simulink subsystem "BAM_Controller"  (R2026a)
settings: Solver=VariableStepAuto
undefined symbols (not defined in the file): DiscIntNeverNeededParam, SimIn, SimPar
libraries: simulink x11, starslibMathOperations x2, sharedTrackingLibrary x1, simulink_extras x1, starslibAxisTransformations x1
(part 2 of 3)

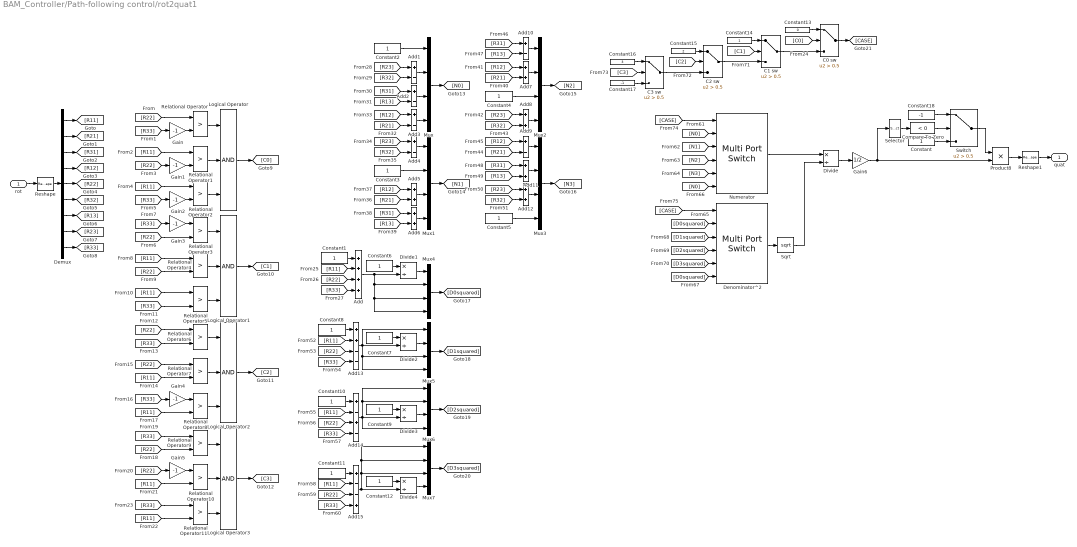
== system BAM_Controller/Path-following control/rot2quat1 ==
  rot : Inport
  Add : Sum  Inputs=++++
  Add{1..4,9..10} (6 alike) : Sum  Inputs=+-
  Add{5..8,11..12} (6 alike) : Sum
  Add13 : Sum  Inputs=++--
  Add14 : Sum  Inputs=+-+-
  Add15 : Sum  Inputs=+--+
  C0 sw : Switch  Criteria=u2 > Threshold  Threshold=0.5  SaturateOnIntegerOverflow=off  InputSameDT=off
  C1 sw : Switch  Criteria=u2 > Threshold  Threshold=0.5  SaturateOnIntegerOverflow=off  InputSameDT=off
  C2 sw : Switch  Criteria=u2 > Threshold  Threshold=0.5  SaturateOnIntegerOverflow=off  InputSameDT=off
  C3 sw : Switch  Criteria=u2 > Threshold  Threshold=0.5  SaturateOnIntegerOverflow=off  InputSameDT=off
  Compare To Zero : simulink/Logic and Bit Operations/Compare To Zero  relop=<  OutDataTypeStr=boolean
  Constant{,1..12,14} (14 alike) : Constant
  Constant13 : Constant  Value=0
  Constant15 : Constant  Value=2
  Constant16 : Constant  Value=3
  Constant17 : Constant  Value=-1
  Constant18 : Constant  Value=-1
  Demux : Demux  Outputs=9
  Denominator^2 : MultiPortSwitch  DataPortOrder=Zero-based contiguous  Inputs=4  DataPortForDefault=Additional data port  zeroidx=on  SaturateOnIntegerOverflow=off  InputSameDT=off
  Divide{,1..4} (5 alike) : Product  Inputs=*/
  Gain{,1..5} (6 alike) : Gain  Gain=-1
  Gain6 : Gain  Gain=1/2
  Logical Operator{,1..3} (4 alike) : Logic  Inputs=3  AllPortsSameDT=off  OutDataTypeStr=boolean
  Mux{,1..7} (8 alike) : Mux
  Numerator : MultiPortSwitch  DataPortOrder=Zero-based contiguous  Inputs=4  DataPortForDefault=Additional data port  zeroidx=on  SaturateOnIntegerOverflow=off  InputSameDT=off
  Product8 : Product
  Relational Operator{,1..11} (12 alike) : RelationalOperator  Operator=>  OutDataTypeStr=boolean  RndMeth=Simplest  InputSameDT=off
  Reshape : Reshape  OutputDimensionality=Column vector (2-D)
  Reshape1 : Reshape  OutputDimensionality=Column vector (2-D)
  Selector : Selector  InputPortWidth=4  IndexOptions=Index vector (dialog)  Indices=1  OutputSizes=1
  Sqrt : Sqrt
  Switch : Switch  Criteria=u2 > Threshold  Threshold=0.5  SaturateOnIntegerOverflow=off  InputSameDT=off
  quat : Outport  VectorParamsAs1DForOutWhenUnconnected=off
  wires:
  Product8/1 -> Reshape1/1
  Reshape1/1 -> quat/1
  Selector/1 -> Compare To Zero/1
  Compare To Zero/1 -> Switch/2
  Constant18/1 -> Switch/1
  Constant/1 -> Switch/3
  Switch/1 -> Product8/1
  [R23] -> Add1/1
  Add/1 -> Divide1/2, Mux4/2, Mux4/3, Mux4/4
  Divide1/1 -> Mux4/1
  Divide2/1 -> Mux5/2
  [N0] -> Numerator/6
  C2 sw/1 -> C1 sw/3
  Constant6/1 -> Divide1/1
  [R12] -> Add7/1
  Constant17/1 -> C3 sw/3
  [N3] -> Numerator/5
  Mux1/1 -> [N1]
  Add7/1 -> Mux2/2
  [N0] -> Numerator/2
  Constant14/1 -> C1 sw/1
  [R21] -> Add3/2
  [R21] -> Add7/2
  [R12] -> Add5/1
  Gain3/1 -> Relational Operator3/1
  Gain5/1 -> Relational Operator10/1
  [R33] -> Relational Operator9/1
  Relational Operator10/1 -> Logical Operator3/2
  Denominator^2/1 -> Sqrt/1
  [R33] -> Gain/1
  Logical Operator/1 -> [C0]
  [R11] -> Relational Operator5/1
  [R11] -> Relational Operator4/1
  [R22] -> Relational Operator/1
  Demux/6 -> [R32]
  Relational Operator4/1 -> Logical Operator1/2
  Relational Operator2/1 -> Logical Operator/3
  [R33] -> Relational Operator5/2
  [R22] -> Relational Operator9/2
  [R22] -> Relational Operator4/2
  Relational Operator9/1 -> Logical Operator3/1
  Demux/4 -> [R12]
  Demux/3 -> [R31]
  Relational Operator5/1 -> Logical Operator1/3
  Numerator/1 -> Divide/1
  Gain4/1 -> Relational Operator8/1
  Divide/1 -> Gain6/1
  Relational Operator8/1 -> Logical Operator2/3
  [R11] -> Relational Operator2/1
  Relational Operator/1 -> Logical Operator/1
  [R33] -> Gain4/1
  [R22] -> Relational Operator3/2
  Gain1/1 -> Relational Operator1/2
  Relational Operator1/1 -> Logical Operator/2
  Reshape/1 -> Demux/1
  [R33] -> Gain3/1
  Demux/5 -> [R22]
  Demux/8 -> [R23]
  C1 sw/1 -> C0 sw/3
  Constant13/1 -> C0 sw/1
  Divide4/1 -> Mux7/4
  Constant4/1 -> Mux2/3
  [D2squared] -> Denominator^2/4
  [R32] -> Add12/2
  [R23] -> Add12/1
  Sqrt/1 -> Divide/2
  [R13] -> Add2/2
  Demux/1 -> [R11]
  Relational Operator3/1 -> Logical Operator1/1
  Demux/2 -> [R21]
  Add12/1 -> Mux3/3
  [R11] -> Relational Operator11/2
  Relational Operator11/1 -> Logical Operator3/3
  [R22] -> Gain5/1
  [R33] -> Gain2/1
  [R11] -> Relational Operator10/2
  Logical Operator1/1 -> [C1]
  Logical Operator2/1 -> [C2]
  [R33] -> Relational Operator6/2
  [R33] -> Relational Operator11/1
  [R22] -> Relational Operator6/1
  [R32] -> Add4/2
  [R22] -> Gain1/1
  [R23] -> Add4/1
  [CASE] -> Denominator^2/1
  Add4/1 -> Mux1/1
  Relational Operator6/1 -> Logical Operator2/1
  [D0squared] -> Denominator^2/2
  Demux/9 -> [R33]
  [D1squared] -> Denominator^2/3
  [R11] -> Add15/2
  Mux2/1 -> [N2]
  Demux/7 -> [R13]
  Constant11/1 -> Add15/1
  [R11] -> Relational Operator7/2
  Logical Operator3/1 -> [C3]
  Mux7/1 -> [D3squared]
  [D3squared] -> Denominator^2/5
  [R11] -> Relational Operator8/2
  [R22] -> Relational Operator7/1
  Gain/1 -> Relational Operator/2
  [R33] -> Add15/4
  [R22] -> Add15/3
  Constant12/1 -> Divide4/1
  [R22] -> Add/3
  Constant3/1 -> Mux1/2
  [R11] -> Relational Operator1/1
  Relational Operator7/1 -> Logical Operator2/2
  [R12] -> Add3/1
  Add6/1 -> Mux1/4
  Add3/1 -> Mux/4
  [R13] -> Add6/2
  [R31] -> Add6/1
  [N1] -> Numerator/3
  rot/1 -> Reshape/1
  Mux4/1 -> [D0squared]
  Gain2/1 -> Relational Operator2/2
  [C0] -> C0 sw/2
  [C2] -> C2 sw/2
  C3 sw/1 -> C2 sw/3
  Constant16/1 -> C3 sw/1
  Constant15/1 -> C2 sw/1
  Divide3/1 -> Mux6/3
  Add15/1 -> Divide4/2, Mux7/3, Mux7/2, Mux7/1
  [CASE] -> Numerator/1
  Constant9/1 -> Divide3/1
  [R11] -> Add13/2
  [R11] -> Add14/2
  Add1/1 -> Mux/2
  Add14/1 -> Divide3/2, Mux6/4, Mux6/2, Mux6/1
  Mux6/1 -> [D2squared]
  [R22] -> Add14/3
  [R22] -> Add13/3
  [R33] -> Add14/4
  [R33] -> Add/4
  Constant10/1 -> Add14/1
  [R32] -> Add1/2
  Mux/1 -> [N0]
  Constant8/1 -> Add13/1
  [R33] -> Add13/4
  [R11] -> Add/2
  C0 sw/1 -> [CASE]
  Add10/1 -> Mux2/1
  [R13] -> Add10/2
  [R21] -> Add5/2
  [C3] -> C3 sw/2
  Add5/1 -> Mux1/3
  [R31] -> Add2/1
  [R31] -> Add10/1
  [N2] -> Numerator/4
  Constant7/1 -> Divide2/1
  Mux5/1 -> [D1squared]
  [D0squared] -> Denominator^2/6
  Add13/1 -> Divide2/2, Mux5/1, Mux5/3, Mux5/4
  [R21] -> Add9/2
  [C1] -> C1 sw/2
  Gain6/1 -> Selector/1, Product8/2
  Constant2/1 -> Mux/1
  Add9/1 -> Mux3/1
  [R12] -> Add9/1
  [R32] -> Add8/2
  Add8/1 -> Mux2/4
  Add11/1 -> Mux3/2
  [R13] -> Add11/2
  Mux3/1 -> [N3]
  Add2/1 -> Mux/3
  [R23] -> Add8/1
  Constant1/1 -> Add/1
  Constant5/1 -> Mux3/4
  [R31] -> Add11/1

== system BAM_Controller/PI&FF Rate Controller/Gain Kff/Diagonalize Vector ==
  Vector : Inport
  Constant2 : Constant  Value=0
  Demux : Demux  Outputs=3
  Reshape (9) to [3x3] column-major : Reshape  OutputDimensionality=Customize  OutputDimensions=[3,3]
  Vector Concatenate : Concatenate  NumInputs=9
  Matrix : Outport  VectorParamsAs1DForOutWhenUnconnected=off
  wires:
  Demux/3 -> Vector Concatenate/9
  Demux/2 -> Vector Concatenate/5
  Vector Concatenate/1 -> Reshape (9) to [3x3] column-major/1
  Reshape (9) to [3x3] column-major/1 -> Matrix/1
  Demux/1 -> Vector Concatenate/1
  Constant2/1 -> Vector Concatenate/3, Vector Concatenate/4, Vector Concatenate/6, Vector Concatenate/7, Vector Concatenate/8, Vector Concatenate/2
  Vector/1 -> Demux/1

== system BAM_Controller/PI&FF Rate Controller/Gain Ki/Diagonalize Vector ==
  Vector : Inport
  Constant2 : Constant  Value=0
  Demux : Demux  Outputs=3
  Reshape (9) to [3x3] column-major : Reshape  OutputDimensionality=Customize  OutputDimensions=[3,3]
  Vector Concatenate : Concatenate  NumInputs=9
  Matrix : Outport  VectorParamsAs1DForOutWhenUnconnected=off
  wires:
  Demux/3 -> Vector Concatenate/9
  Demux/2 -> Vector Concatenate/5
  Vector Concatenate/1 -> Reshape (9) to [3x3] column-major/1
  Reshape (9) to [3x3] column-major/1 -> Matrix/1
  Demux/1 -> Vector Concatenate/1
  Constant2/1 -> Vector Concatenate/3, Vector Concatenate/4, Vector Concatenate/6, Vector Concatenate/7, Vector Concatenate/8, Vector Concatenate/2
  Vector/1 -> Demux/1

== system BAM_Controller/PI&FF Rate Controller/Gain Kp/Diagonalize Vector ==
  Vector : Inport
  Constant2 : Constant  Value=0
  Demux : Demux  Outputs=3
  Reshape (9) to [3x3] column-major : Reshape  OutputDimensionality=Customize  OutputDimensions=[3,3]
  Vector Concatenate : Concatenate  NumInputs=9
  Matrix : Outport  VectorParamsAs1DForOutWhenUnconnected=off
  wires:
  Demux/3 -> Vector Concatenate/9
  Demux/2 -> Vector Concatenate/5
  Vector Concatenate/1 -> Reshape (9) to [3x3] column-major/1
  Reshape (9) to [3x3] column-major/1 -> Matrix/1
  Demux/1 -> Vector Concatenate/1
  Constant2/1 -> Vector Concatenate/3, Vector Concatenate/4, Vector Concatenate/6, Vector Concatenate/7, Vector Concatenate/8, Vector Concatenate/2
  Vector/1 -> Demux/1

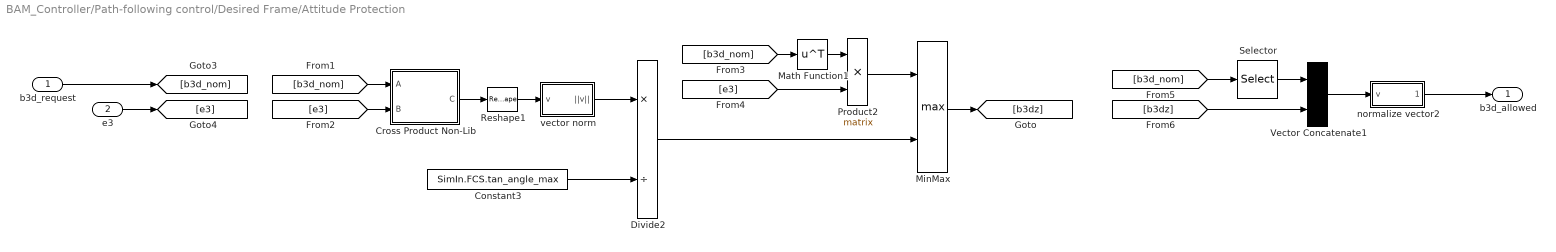
== system BAM_Controller/Path-following control/Desired Frame/Attitude Protection ==
  b3d_request : Inport
  e3 : Inport  Port=2
  Constant3 : Constant  Value=SimIn.FCS.tan_angle_max
  Cross Product Non-Lib : Subsystem
  Divide2 : Product  Inputs=*/
  Math Function1 : Math  Operator=transpose  SignedPower=on
  MinMax : MinMax  Function=max  Inputs=2
  Product2 : Product  Multiplication=Matrix(*)
  Reshape1 : Reshape  OutputDimensionality=Column vector (2-D)
  Selector : Selector  InputPortWidth=3  IndexOptions=Index vector (dialog)  Indices=[1 2]  OutputSizes=1
  Vector Concatenate1 : Concatenate  Mode=Multidimensional array
  normalize vector2 : Subsystem
  vector norm : Subsystem
  b3d_allowed : Outport  VectorParamsAs1DForOutWhenUnconnected=off
  wires:
  MinMax/1 -> [b3dz]
  [e3] -> Product2/2
  Divide2/1 -> MinMax/2
  Product2/1 -> MinMax/1
  Constant3/1 -> Divide2/2
  [e3] -> Cross Product Non-Lib/2(B)
  [b3d_nom] -> Cross Product Non-Lib/1(A)
  Reshape1/1 -> vector norm/1(v)
  vector norm/1(||v||) -> Divide2/1
  normalize vector2/1(v / ||v||) -> b3d_allowed/1
  Cross Product Non-Lib/1(C) -> Reshape1/1
  [b3d_nom] -> Selector/1
  Selector/1 -> Vector Concatenate1/1
  Vector Concatenate1/1 -> normalize vector2/1(v)
  [b3dz] -> Vector Concatenate1/2
  b3d_request/1 -> [b3d_nom]
  e3/1 -> [e3]
  Math Function1/1 -> Product2/1
  [b3d_nom] -> Math Function1/1

== system BAM_Controller/Path-following control/Desired Frame/Cross Product Non-Lib ==
  A : Inport
  B : Inport  Port=2
  Subsystem : Subsystem
  Subsystem1 : Subsystem
  Sum : Sum  Inputs=+|-  InputSameDT=on  SaturateOnIntegerOverflow=on  OutDataTypeStr=Inherit: Same as first input
  C : Outport  VectorParamsAs1DForOutWhenUnconnected=off
  wires:
  Subsystem/1(Out1) -> Sum/1
  B/1 -> Subsystem/2(B), Subsystem1/2(B)
  Subsystem1/1(Out1) -> Sum/2
  A/1 -> Subsystem/1(A), Subsystem1/1(A)
  Sum/1 -> C/1

== system BAM_Controller/Path-following control/Desired Frame/DLPF ==
  In1 : Inport
  Constant1 : Constant  Value=0
  Discrete-Time Integrator1 : DiscreteIntegrator  gainval=1  ExternalReset=either  InitialConditionSource=external  SampleTime=SimIn.FCS.t_control  UpperSaturationLimit=1  LowerSaturationLimit=0  ICPrevOutput=DiscIntNeverNeededParam  ICPrevScaledInput=DiscIntNeverNeededParam
  Gain : Gain  Gain=w
  Sum : Sum  Inputs=|+-
  Out1 : Outport  VectorParamsAs1DForOutWhenUnconnected=off
  wires:
  In1/1 -> Discrete-Time Integrator1/3, Sum/1
  Sum/1 -> Gain/1
  Discrete-Time Integrator1/1 -> Out1/1, Sum/2
  Constant1/1 -> Discrete-Time Integrator1/2
  Gain/1 -> Discrete-Time Integrator1/1

== system BAM_Controller/Path-following control/Desired Frame/DLPF1 ==
  In1 : Inport
  Constant1 : Constant  Value=0
  Discrete-Time Integrator1 : DiscreteIntegrator  gainval=1  ExternalReset=either  InitialConditionSource=external  SampleTime=SimIn.FCS.t_control  UpperSaturationLimit=1  LowerSaturationLimit=0  ICPrevOutput=DiscIntNeverNeededParam  ICPrevScaledInput=DiscIntNeverNeededParam
  Gain : Gain  Gain=w
  Sum : Sum  Inputs=|+-
  Out1 : Outport  VectorParamsAs1DForOutWhenUnconnected=off
  wires:
  Gain/1 -> Discrete-Time Integrator1/1
  Constant1/1 -> Discrete-Time Integrator1/2
  Discrete-Time Integrator1/1 -> Sum/2, Out1/1
  Sum/1 -> Gain/1
  In1/1 -> Sum/1, Discrete-Time Integrator1/3

== system BAM_Controller/Path-following control/Desired Frame/normalize vector1 ==
  v : Inport
  Add : Sum
  Compare To Constant : simulink/Logic and Bit Operations/Compare To Constant  relop===  const=0  OutDataTypeStr=boolean
  Constant : Constant
  Constant1 : Constant  Value=0
  Divide3 : Product  Inputs=*/
  Switch : Switch  Criteria=u2 > Threshold  Threshold=0.5  SaturateOnIntegerOverflow=off  InputSameDT=off
  vector norm : Subsystem
  v / ||v|| : Outport  VectorParamsAs1DForOutWhenUnconnected=off
  wires:
  Divide3/1 -> v / ||v||/1
  vector norm/1(||v||) -> Compare To Constant/1, Add/1
  v/1 -> vector norm/1(v), Divide3/1
  Add/1 -> Divide3/2
  Switch/1 -> Add/2
  Compare To Constant/1 -> Switch/2
  Constant/1 -> Switch/1
  Constant1/1 -> Switch/3

== system BAM_Controller/Path-following control/Desired Frame/normalize vector2 ==
  v : Inport
  Add : Sum
  Compare To Constant : simulink/Logic and Bit Operations/Compare To Constant  relop===  const=0  OutDataTypeStr=boolean
  Constant : Constant
  Constant1 : Constant  Value=0
  Divide3 : Product  Inputs=*/
  Switch : Switch  Criteria=u2 > Threshold  Threshold=0.5  SaturateOnIntegerOverflow=off  InputSameDT=off
  vector norm : Subsystem
  v / ||v|| : Outport  VectorParamsAs1DForOutWhenUnconnected=off
  wires:
  Constant1/1 -> Switch/3
  Constant/1 -> Switch/1
  Compare To Constant/1 -> Switch/2
  Switch/1 -> Add/2
  Add/1 -> Divide3/2
  v/1 -> Divide3/1, vector norm/1(v)
  vector norm/1(||v||) -> Add/1, Compare To Constant/1
  Divide3/1 -> v / ||v||/1

== system BAM_Controller/Path-following control/Path/DLPF7 ==
  x : Inport
  Discrete-Time Integrator : DiscreteIntegrator  InitialConditionSource=external  SampleTime=-1  ICPrevOutput=DiscIntNeverNeededParam  ICPrevScaledInput=DiscIntNeverNeededParam
  Gain : Gain  Gain=bw
  Sum : Sum  Inputs=-+|
  xf : Outport  VectorParamsAs1DForOutWhenUnconnected=off
  wires:
  x/1 -> Discrete-Time Integrator/2, Sum/2
  Sum/1 -> Gain/1
  Gain/1 -> Discrete-Time Integrator/1
  Discrete-Time Integrator/1 -> Sum/1, xf/1

== system BAM_Controller/Path-following control/Path/DLPF8 ==
  x : Inport
  Discrete-Time Integrator : DiscreteIntegrator  InitialConditionSource=external  SampleTime=-1  ICPrevOutput=DiscIntNeverNeededParam  ICPrevScaledInput=DiscIntNeverNeededParam
  Gain : Gain  Gain=bw
  Sum : Sum  Inputs=-+|
  xf : Outport  VectorParamsAs1DForOutWhenUnconnected=off
  wires:
  Discrete-Time Integrator/1 -> xf/1, Sum/1
  Gain/1 -> Discrete-Time Integrator/1
  Sum/1 -> Gain/1
  x/1 -> Sum/2, Discrete-Time Integrator/2

== system BAM_Controller/Path-following control/Path/Heading Hold Logic prevents badness when trajectory is vertical ==
  quat : Inport
  tangent : Inport  Port=2
  Constant1 : Constant  Value=SimIn.FCS.e3
  Constant3 : Constant  Value=0.05
  Cross Product1 : starslibMathOperations/Cross Product
  Heading Vector in Horz Plane : Subsystem
  Relational Operator : RelationalOperator  Operator=>  OutDataTypeStr=boolean  RndMeth=Simplest  InputSameDT=off
  Vector Norm : Subsystem  mask(Vector Norm){}
      mask help: Calculates the 2-norm of the input vector.
      settings: CopyFcn=set_param(gcb,'LinkStatus','none')
  tangentDes3 : Switch  Criteria=u2 > Threshold  Threshold=0.5  SaturateOnIntegerOverflow=off  InputSameDT=off
  t_F : Outport  VectorParamsAs1DForOutWhenUnconnected=off
  wires:
  Relational Operator/1 -> tangentDes3/2
  [headingVector] -> tangentDes3/3
  Constant3/1 -> Relational Operator/2
  Vector Norm/1(||v||) -> Relational Operator/1
  Constant1/1 -> Cross Product1/2
  Cross Product1/1 -> Vector Norm/1(v)
  tangent/1 -> tangentDes3/1, Cross Product1/1
  tangentDes3/1 -> t_F/1
  Heading Vector in Horz Plane/1(headVec) -> [headingVector]
  quat/1 -> Heading Vector in Horz Plane/1(quat)

== system BAM_Controller/Path-following control/Path/normalize vector2 ==
  v : Inport
  Add : Sum
  Compare To Constant : simulink/Logic and Bit Operations/Compare To Constant  relop===  const=0  OutDataTypeStr=boolean
  Constant : Constant
  Constant1 : Constant  Value=0
  Divide3 : Product  Inputs=*/
  Switch : Switch  Criteria=u2 > Threshold  Threshold=0.5  SaturateOnIntegerOverflow=off  InputSameDT=off
  vector norm : Subsystem
  v / ||v|| : Outport  VectorParamsAs1DForOutWhenUnconnected=off
  wires:
  Divide3/1 -> v / ||v||/1
  vector norm/1(||v||) -> Compare To Constant/1, Add/1
  v/1 -> vector norm/1(v), Divide3/1
  Add/1 -> Divide3/2
  Switch/1 -> Add/2
  Compare To Constant/1 -> Switch/2
  Constant/1 -> Switch/1
  Constant1/1 -> Switch/3

== system BAM_Controller/Path-following control/f_c/prevent div by 0 ==
  In1 : Inport
  Compare To Zero : simulink/Logic and Bit Operations/Compare To Zero  relop=~=  OutDataTypeStr=boolean
  Constant : Constant
  Switch : Switch  Criteria=u2 > Threshold  SaturateOnIntegerOverflow=off  InputSameDT=off
  Out1 : Outport  VectorParamsAs1DForOutWhenUnconnected=off
  wires:
  Switch/1 -> Out1/1
  Constant/1 -> Switch/3
  Compare To Zero/1 -> Switch/2
  In1/1 -> Switch/1, Compare To Zero/1

== system BAM_Controller/Path-following control/omega_c/Subsystem ==
  function : TriggerPort  TriggerType=function-call  VariantControl=(inherit)
  From : From  Commented=on  GotoTag=Rtilde
  Gain2 : Gain  Commented=on  Gain=SimIn.FCS.r2d
  MATLAB Function : MATLAB Function  Commented=on  TreatAsAtomicUnit=on
  desired frame error : Scope  Commented=on
      settings: SampleTime=FCS.t_control  ActiveDisplayYMinimum=-0.00376  ActiveDisplayYMaximum=0.00938  DataLoggingVariableName=ScopeData2
  wires:
  Gain2/1 -> desired frame error/1
  From/1 -> MATLAB Function/1(R)
  MATLAB Function/1(rpy) -> Gain2/1

== system BAM_Controller/Path-following control/Desired Frame/Attitude Protection/Cross Product Non-Lib ==
  A : Inport
  B : Inport  Port=2
  Subsystem : Subsystem
  Subsystem1 : Subsystem
  Sum : Sum  Inputs=+|-  InputSameDT=on  SaturateOnIntegerOverflow=on  OutDataTypeStr=Inherit: Same as first input
  C : Outport  VectorParamsAs1DForOutWhenUnconnected=off
  wires:
  Subsystem/1(Out1) -> Sum/1
  B/1 -> Subsystem/2(B), Subsystem1/2(B)
  Subsystem1/1(Out1) -> Sum/2
  A/1 -> Subsystem/1(A), Subsystem1/1(A)
  Sum/1 -> C/1

== system BAM_Controller/Path-following control/Desired Frame/Attitude Protection/normalize vector2 ==
  v : Inport
  Add : Sum
  Compare To Constant : simulink/Logic and Bit Operations/Compare To Constant  relop===  const=0  OutDataTypeStr=boolean
  Constant : Constant
  Constant1 : Constant  Value=0
  Divide3 : Product  Inputs=*/
  Switch : Switch  Criteria=u2 > Threshold  Threshold=0.5  SaturateOnIntegerOverflow=off  InputSameDT=off
  vector norm : Subsystem
  v / ||v|| : Outport  VectorParamsAs1DForOutWhenUnconnected=off
  wires:
  Constant1/1 -> Switch/3
  Constant/1 -> Switch/1
  Compare To Constant/1 -> Switch/2
  Switch/1 -> Add/2
  Add/1 -> Divide3/2
  v/1 -> Divide3/1, vector norm/1(v)
  vector norm/1(||v||) -> Add/1, Compare To Constant/1
  Divide3/1 -> v / ||v||/1

== system BAM_Controller/Path-following control/Desired Frame/Attitude Protection/vector norm ==
  v : Inport
  Abs3 : Abs  SaturateOnIntegerOverflow=off
  Math Function1 : Math  Operator=transpose  SignedPower=on
  Matrix Multiply1 : Product  Multiplication=Matrix(*)
  Reshape7 : Reshape  OutputDimensionality=Column vector (2-D)
  Sqrt3 : Sqrt
  ||v|| : Outport  VectorParamsAs1DForOutWhenUnconnected=off
  wires:
  Sqrt3/1 -> ||v||/1
  Abs3/1 -> Sqrt3/1
  v/1 -> Reshape7/1
  Matrix Multiply1/1 -> Abs3/1
  Math Function1/1 -> Matrix Multiply1/1
  Reshape7/1 -> Matrix Multiply1/2, Math Function1/1

== system BAM_Controller/Path-following control/Desired Frame/Cross Product Non-Lib/Subsystem ==
  A : Inport
  B : Inport  Port=2
  Demux : Demux  Outputs=3
  Demux1 : Demux  Outputs=3
  Mux : Mux  Inputs=3
  i x j : Product  InputSameDT=on  SaturateOnIntegerOverflow=on  OutDataTypeStr=Inherit: Same as first input
  j x k : Product  InputSameDT=on  SaturateOnIntegerOverflow=on  OutDataTypeStr=Inherit: Same as first input
  k x i : Product  InputSameDT=on  SaturateOnIntegerOverflow=on  OutDataTypeStr=Inherit: Same as first input
  Out1 : Outport  VectorParamsAs1DForOutWhenUnconnected=off
  wires:
  Demux1/3 -> j x k/2
  i x j/1 -> Mux/3
  Demux/3 -> k x i/1
  Mux/1 -> Out1/1
  Demux/1 -> i x j/1
  A/1 -> Demux/1
  j x k/1 -> Mux/1
  Demux1/1 -> k x i/2
  B/1 -> Demux1/1
  k x i/1 -> Mux/2
  Demux1/2 -> i x j/2
  Demux/2 -> j x k/1

== system BAM_Controller/Path-following control/Desired Frame/Cross Product Non-Lib/Subsystem1 ==
  A : Inport
  B : Inport  Port=2
  Demux : Demux  Outputs=3
  Demux1 : Demux  Outputs=3
  Mux : Mux  Inputs=3
  i x k : Product  InputSameDT=on  SaturateOnIntegerOverflow=on  OutDataTypeStr=Inherit: Same as first input
  j x i : Product  InputSameDT=on  SaturateOnIntegerOverflow=on  OutDataTypeStr=Inherit: Same as first input
  k x j : Product  InputSameDT=on  SaturateOnIntegerOverflow=on  OutDataTypeStr=Inherit: Same as first input
  Out1 : Outport  VectorParamsAs1DForOutWhenUnconnected=off
  wires:
  Demux/1 -> i x k/1
  A/1 -> Demux/1
  j x i/1 -> Mux/3
  Demux1/3 -> i x k/2
  k x j/1 -> Mux/1
  Demux1/1 -> j x i/2
  B/1 -> Demux1/1
  Demux/3 -> k x j/1
  Demux/2 -> j x i/1
  Mux/1 -> Out1/1
  i x k/1 -> Mux/2
  Demux1/2 -> k x j/2

== system BAM_Controller/Path-following control/Desired Frame/normalize vector1/vector norm ==
  v : Inport
  Abs3 : Abs  SaturateOnIntegerOverflow=off
  Math Function1 : Math  Operator=transpose  SignedPower=on
  Matrix Multiply1 : Product  Multiplication=Matrix(*)
  Reshape7 : Reshape  OutputDimensionality=Column vector (2-D)
  Sqrt3 : Sqrt
  ||v|| : Outport  VectorParamsAs1DForOutWhenUnconnected=off
  wires:
  Sqrt3/1 -> ||v||/1
  v/1 -> Reshape7/1
  Matrix Multiply1/1 -> Abs3/1
  Math Function1/1 -> Matrix Multiply1/1
  Abs3/1 -> Sqrt3/1
  Reshape7/1 -> Matrix Multiply1/2, Math Function1/1

== system BAM_Controller/Path-following control/Desired Frame/normalize vector2/vector norm ==
  v : Inport
  Abs3 : Abs  SaturateOnIntegerOverflow=off
  Math Function1 : Math  Operator=transpose  SignedPower=on
  Matrix Multiply1 : Product  Multiplication=Matrix(*)
  Reshape7 : Reshape  OutputDimensionality=Column vector (2-D)
  Sqrt3 : Sqrt
  ||v|| : Outport  VectorParamsAs1DForOutWhenUnconnected=off
  wires:
  Reshape7/1 -> Math Function1/1, Matrix Multiply1/2
  Abs3/1 -> Sqrt3/1
  Math Function1/1 -> Matrix Multiply1/1
  Matrix Multiply1/1 -> Abs3/1
  v/1 -> Reshape7/1
  Sqrt3/1 -> ||v||/1

== system BAM_Controller/Path-following control/Path/Heading Hold Logic prevents badness when trajectory is vertical/Heading Vector in Horz Plane ==
  quat : Inport
  1st Col : Selector  NumberOfDimensions=2  InputPortWidth=3  IndexOptions=Select all,Index vector (dialog)  Indices=[1 3],1  OutputSizes=1,1
  MATLAB Function : MATLAB Function  TreatAsAtomicUnit=on
  MATLAB Function1 : MATLAB Function  TreatAsAtomicUnit=on
  MATLAB Function4 : MATLAB Function  TreatAsAtomicUnit=on
  Math Function6 : Math  Operator=transpose  SignedPower=on
  "Subtract phi, theta" : Gain  Gain=[1;1;0]
  Sum1 : Sum  Inputs=|+-
  headVec : Outport  VectorParamsAs1DForOutWhenUnconnected=off
  wires:
  1st Col/1 -> headVec/1
  MATLAB Function1/1(euler_output) -> Sum1/1, "Subtract phi, theta"/1
  quat/1 -> MATLAB Function1/1(quat_input)
  "Subtract phi, theta"/1 -> Sum1/2
  Sum1/1 -> MATLAB Function4/1(quat_input)
  Math Function6/1 -> 1st Col/1
  MATLAB Function4/1(quat_output) -> MATLAB Function/1(q)
  MATLAB Function/1(R) -> Math Function6/1

== system BAM_Controller/Path-following control/Path/Heading Hold Logic prevents badness when trajectory is vertical/Vector Norm ==
  v : Inport
  Math Function1 : Math  Operator=transpose  SignedPower=on
  Matrix Multiply1 : Product  Multiplication=Matrix(*)
  Reshape7 : Reshape  OutputDimensionality=Column vector (2-D)
  Sqrt3 : Sqrt
  ||v|| : Outport  VectorParamsAs1DForOutWhenUnconnected=off
  wires:
  Sqrt3/1 -> ||v||/1
  v/1 -> Reshape7/1
  Math Function1/1 -> Matrix Multiply1/1
  Matrix Multiply1/1 -> Sqrt3/1
  Reshape7/1 -> Matrix Multiply1/2, Math Function1/1

== system BAM_Controller/Path-following control/Path/normalize vector2/vector norm ==
  v : Inport
  Abs3 : Abs  SaturateOnIntegerOverflow=off
  Math Function1 : Math  Operator=transpose  SignedPower=on
  Matrix Multiply1 : Product  Multiplication=Matrix(*)
  Reshape7 : Reshape  OutputDimensionality=Column vector (2-D)
  Sqrt3 : Sqrt
  ||v|| : Outport  VectorParamsAs1DForOutWhenUnconnected=off
  wires:
  Sqrt3/1 -> ||v||/1
  v/1 -> Reshape7/1
  Matrix Multiply1/1 -> Abs3/1
  Math Function1/1 -> Matrix Multiply1/1
  Abs3/1 -> Sqrt3/1
  Reshape7/1 -> Matrix Multiply1/2, Math Function1/1

== system BAM_Controller/Path-following control/Desired Frame/Attitude Protection/Cross Product Non-Lib/Subsystem ==
  A : Inport
  B : Inport  Port=2
  Demux : Demux  Outputs=3
  Demux1 : Demux  Outputs=3
  Mux : Mux  Inputs=3
  i x j : Product  InputSameDT=on  SaturateOnIntegerOverflow=on  OutDataTypeStr=Inherit: Same as first input
  j x k : Product  InputSameDT=on  SaturateOnIntegerOverflow=on  OutDataTypeStr=Inherit: Same as first input
  k x i : Product  InputSameDT=on  SaturateOnIntegerOverflow=on  OutDataTypeStr=Inherit: Same as first input
  Out1 : Outport  VectorParamsAs1DForOutWhenUnconnected=off
  wires:
  Demux1/3 -> j x k/2
  i x j/1 -> Mux/3
  Demux/3 -> k x i/1
  Mux/1 -> Out1/1
  Demux/1 -> i x j/1
  A/1 -> Demux/1
  j x k/1 -> Mux/1
  Demux1/1 -> k x i/2
  B/1 -> Demux1/1
  k x i/1 -> Mux/2
  Demux1/2 -> i x j/2
  Demux/2 -> j x k/1

== system BAM_Controller/Path-following control/Desired Frame/Attitude Protection/Cross Product Non-Lib/Subsystem1 ==
  A : Inport
  B : Inport  Port=2
  Demux : Demux  Outputs=3
  Demux1 : Demux  Outputs=3
  Mux : Mux  Inputs=3
  i x k : Product  InputSameDT=on  SaturateOnIntegerOverflow=on  OutDataTypeStr=Inherit: Same as first input
  j x i : Product  InputSameDT=on  SaturateOnIntegerOverflow=on  OutDataTypeStr=Inherit: Same as first input
  k x j : Product  InputSameDT=on  SaturateOnIntegerOverflow=on  OutDataTypeStr=Inherit: Same as first input
  Out1 : Outport  VectorParamsAs1DForOutWhenUnconnected=off
  wires:
  Demux/1 -> i x k/1
  A/1 -> Demux/1
  j x i/1 -> Mux/3
  Demux1/3 -> i x k/2
  k x j/1 -> Mux/1
  Demux1/1 -> j x i/2
  B/1 -> Demux1/1
  Demux/3 -> k x j/1
  Demux/2 -> j x i/1
  Mux/1 -> Out1/1
  i x k/1 -> Mux/2
  Demux1/2 -> k x j/2

== system BAM_Controller/Path-following control/Desired Frame/Attitude Protection/normalize vector2/vector norm ==
  v : Inport
  Abs3 : Abs  SaturateOnIntegerOverflow=off
  Math Function1 : Math  Operator=transpose  SignedPower=on
  Matrix Multiply1 : Product  Multiplication=Matrix(*)
  Reshape7 : Reshape  OutputDimensionality=Column vector (2-D)
  Sqrt3 : Sqrt
  ||v|| : Outport  VectorParamsAs1DForOutWhenUnconnected=off
  wires:
  Reshape7/1 -> Math Function1/1, Matrix Multiply1/2
  Abs3/1 -> Sqrt3/1
  Math Function1/1 -> Matrix Multiply1/1
  Matrix Multiply1/1 -> Abs3/1
  v/1 -> Reshape7/1
  Sqrt3/1 -> ||v||/1

== matlab function BAM_Controller/Path-following control/omega_c/MATLAB Function4 ==
  data: M input; tr output
function tr = trace(M)
%#codegen

tr = trace(M);

== matlab function BAM_Controller/Path-following control/omega_c/Subsystem/MATLAB Function ==
  data: R input; rpy output
function rpy = RotToEuler(R)

p = -asin(R(1,3));
r = atan2(R(2,3),R(3,3));
y = atan2(R(1,2),R(1,1));

rpy = [r p y]';

== matlab function BAM_Controller/Avoidance Planner/Ball is Moving/Collision Assessment ==
  data: time input; FlagMode output; wptVect input; timeVect input; parseVect input; tau input; bb_traj input; clearFlag output; dbRelTraj output; d_traj output; missDist output; currSep output
function [FlagMode, ...
		  clearFlag, ....
		  dbRelTraj, ...
		  d_traj, ...
		  missDist, ...
		  currSep] ...
	  = fcn( ...
		  time, ...
		  wptVect, ...
		  timeVect, ...
		  parseVect, ...
		  tau, ...
		  bb_traj)
% inputs:
	% t_now - sim clock
	% wptVect   \
	% timeVect   |---> Inputs for Bezier function
	% parseVect /
	% EOM - Current drone sensor data
	% tau - time measurement for t_horizon
	% bb_traj - ball trajectory from EKF
% outputs:
	% t_cpa - closest point of approach (debugging)
	% idx - current count from the index (debugging)
	% FlagMode - current flag for the drones state
	% missDist - distance between drone and ball (scalar)
	% dbRelTraj - relative traj of ball IRT drone
	% clearFlag - system to clear flag to nominal given conditions

% ----- Initialize ----- %
b_pos = bb_traj(1:3,:);
b_vel = bb_traj(4:6,:);

Nmax = size(b_pos, 2);
dbRelTraj = zeros(6, Nmax, 'like', b_pos);

% ----- Bezier Functions to path future drone path ----- %

t_query = (time + tau)';
[wptCellArray, timeCellArray] = decodeBezierArray(wptVect, timeVect, parseVect);

[pos_i, vel_i, ~, ~, ~, ~] = evalSegments( ...
    wptCellArray{1}, wptCellArray{2}, wptCellArray{3}, ...
    timeCellArray{1}, timeCellArray{2}, timeCellArray{3}, ...
    t_query);

d_pos = pos_i;
d_vel = vel_i;

% ----- Constants ----- % 
R_safe = 3;
buffer = .75;
tau_delay = .2;
aLatMax = 11;
a_eff = .7 * aLatMax;
N = min(size(d_pos, 2), size(b_pos, 2));

% ----- Resizing ----- %
d_pos = d_pos(:,1:N);
d_vel = d_vel(:,1:N);
d_traj = [d_pos; d_vel];

b_pos = b_pos(:,1:N);
b_vel = b_vel(:,1:N);

tau_use = tau(1:N);

% ----- clearMode Setup ----- %
pos_rel = b_pos - d_pos;
vel_rel = b_vel - d_vel;

dbRelTraj(1:3,1:N) = pos_rel;
dbRelTraj(4:6,1:N) = vel_rel; % 6xN

sep = sqrt(sum(pos_rel .^2, 1));
[missDist, idx] = min(sep);
currSep = sep(1); % Current dist between ball and drone

closing_now = dot(pos_rel(:,1), vel_rel(:,1)) < 0;
diverging_now = dot(pos_rel(:,1), vel_rel(:,1)) >= 0;

R_clear = R_safe + buffer + 0.5;

clearFlag = (diverging_now && sep(1) > R_clear) || ...
            (idx == 1 && diverging_now);

t_cpa = tau_use(idx);

% ----- Multi-factor Flag Requirements ----- %
t_use = max(0, t_cpa - tau_delay); % time available for maneuver after delay
d_need = max(0, (R_safe + buffer) - missDist); % Distance needed to move after buffer
d_avail = .5 * a_eff * t_use ^2; % mx lateral displacement before t_cpa


% ----- Jitter Flag Prevention ----- %
persistent threatLatched onCount offCount

if isempty(threatLatched)
    threatLatched = false;
    onCount = uint8(0);
    offCount = uint8(0);
end

triggerRaw = closing_now && (d_need > 0) && (d_avail <= d_need);
clearRaw = (diverging_now && sep(1) > R_clear) || (idx == 1 && diverging_now);

if triggerRaw
    onCount = onCount + 1;
    offCount = uint8(0);
else
    onCount = uint8(0);
end

if clearRaw
    offCount = offCount + 1;
else
    offCount = uint8(0);
end

if ~threatLatched && onCount >= 3
    threatLatched = true;
end

if threatLatched && offCount >= 3
    threatLatched = false;
end

FlagMode = threatLatched;
clearFlag = ~threatLatched && clearRaw;

== matlab function BAM_Controller/Avoidance Planner/Ball is Moving/EKF Post Processing ==
  data: xhat input size=[6 1]; tau output; bb_traj output; time_now input; vel_est output; xhatx output; xhaty output; xhatz output; bbx output; bby output; bbz output; bbvx output; bbvy output; bbvz output
function [tau, bb_traj, vel_est, xhatx, xhaty, xhatz, bbx, bby, bbz, bbvx, bbvy, bbvz] = buildTraj(xhat, time_now)
% buildTraj
% Predict baseball trajectory from current position and estimated velocity,
% using a forward-Euler integration that includes aerodynamic drag.
%
% Important:
%   This version DOES NOT use xhat(4:6) as velocity.
%   It only trusts xhat(1:3) as position, then estimates velocity from
%   recent position history using estimateBallVelocityFromHistory.m.
%
%   The prediction model includes velocity-opposed quadratic drag to
%   better match the baseball trajectories generated by Dynamics.slx
%   (via Create_BBall_Traj.m), which use drag coefficients in [0.2, 0.4],
%   Magnus spin forces (1600-2600 RPM), and randomized gravity (0.6g-1.0g).
%   We model drag here but NOT Magnus force, since estimating the spin
%   axis from noisy position data is not tractable. Drag is the dominant
%   deceleration effect; Magnus causes lateral curvature but is smaller
%   in magnitude. This is a known and defensible simplification.
%
% Startup Guard:
%   When the "Ball is Moving" action subsystem first activates, the EKF
%   block's internal state initializes to zero before converging to real
%   measurements. This causes a transient where xhat jumps from [0;0;0]
%   to the actual ball position. If the velocity estimator sees that jump
%   in its history buffer, it computes an enormous (incorrect) velocity.
%   To prevent this, we count samples since activation and suppress
%   velocity estimation until enough clean samples have accumulated in
%   the history buffer (min_samples = N_hist + 10). During the guard
%   window, the ball is predicted as stationary at its current position.
%
% Inputs
%   xhat     : state vector with position in xhat(1:3)
%   time_now : current time in seconds
%
% Internal parameters (set in opts struct below):
%   opts.dt          = prediction timestep, default 1/200 (200 Hz)
%   opts.t_horizon   = prediction horizon in seconds, default 6
%   opts.g           = gravity magnitude, default 9.81 m/s^2
%   opts.N_hist      = velocity history samples, default 100
%   opts.speed_clip  = velocity clip in m/s, default 60
%   opts.verbose     = print debug info, default false
%
% Outputs
%   tau      : 1xN future relative times (seconds from now)
%   bb_traj  : 6xN [x;y;z;vx;vy;vz] predicted ball trajectory
%   vel_est  : 3x1 estimated initial velocity at current time
%   xhatx    : scalar, current x position used (debug)
%   xhaty    : scalar, current y position used (debug)
%   xhatz    : scalar, current z position used (debug)
%   bbx      : scalar, predicted x at 1s ahead (debug, index 200)
%   bby      : scalar, predicted y at 1s ahead (debug, index 200)
%   bbz      : scalar, predicted z at 1s ahead (debug, index 200)
%   bbvx     : scalar, predicted vx at 1s ahead (debug)
%   bbvy     : scalar, predicted vy at 1s ahead (debug)
%   bbvz     : scalar, predicted vz at 1s ahead (debug)

%% ======================== Configuration ================================

% --- Prediction parameters ---
opts.dt        = 1/200;    % prediction timestep (s), matches sim rate
opts.t_horizon = 3;        % prediction horizon (s), covers full ball flight
opts.g         = 9.81;     % gravity magnitude (m/s^2)
opts.N_hist    = 10;      % number of position samples for velocity estimation
opts.speed_clip = 60;      % maximum plausible ball speed (m/s), clips outliers
opts.verbose   = false;    % set true to print debug info to command window

% Precompute the drag deceleration coefficient:
%   F_drag = 0.5 * rho * Cd * A * |v|^2  (opposing velocity)
%   a_drag = F_drag / m = drag_coeff * |v|^2
% In the Euler loop below this is applied as: a_drag_vec = -drag_coeff * speed * vel
% which gives the correct magnitude and direction (opposing velocity).
drag_coeff = 0.00540023495;

% --- Gravity vector ---
% BAM convention note: The original buildTraj used z-up convention
% (z0 + vz*t - 0.5*g*t^2). We preserve that here. In NED (z-down),
% gravity adds to z; in z-up, gravity subtracts. Ensure this matches
% whatever convention the EKF and Collision Assessment expect.
% If your system is NED (z-positive-down), change to [0; 0; +opts.g].
g_vec = [0; 0; -opts.g];  % z-up: gravity pulls downward (negative z)

%% =================== Startup Guard (Persistent) ========================

% Track how many samples have elapsed since the action subsystem activated.
% This persistent variable resets when the MATLAB Function block
% re-initializes (i.e., when "Ball is Moving" activates for the first time
% or after a model reset). It does NOT reset if the action subsystem
% merely deactivates and reactivates with states held — check the
% Action Port "States when re-enabled" setting if you see transients
% on re-entry.
persistent sample_count
if isempty(sample_count)
    sample_count = int32(0);
end
sample_count = sample_count + int32(1);

%% =================== Compute Prediction Horizon =======================

N_horizon = round(opts.t_horizon / opts.dt) + 1;

%% =================== Default Output Initialization =====================
% All outputs must be assigned before any early return to satisfy
% MATLAB Coder (Simulink code generation). Uninitialized outputs on
% any code path will cause a build error.

tau     = zeros(1, N_horizon);
bb_traj = zeros(6, N_horizon);
vel_est = zeros(3, 1);
xhatx = 0; xhaty = 0; xhatz = 0;
bbx = 0;   bby = 0;   bbz = 0;
bbvx = 0;  bbvy = 0;  bbvz = 0;

%% =================== Input Validation ==================================

if numel(xhat) < 3
    % Cannot proceed without at least [x; y; z]. Return default zeros.
    % Using error() here would crash the sim; returning zeros lets
    % downstream blocks handle it gracefully (Collision Assessment
    % will see no threat).
    return;
end

%% =================== Extract Current Position ==========================

pos_now = xhat(1:3);

%% =================== Velocity Estimation ===============================
% Estimate velocity from recent position history using polynomial fitting.
%
% Guard logic: During the first min_samples timesteps after activation,
% the velocity estimator's history buffer contains zero-init garbage from
% the EKF's cold start. Using that data would produce enormous (wrong)
% velocities due to the step from [0,0,0] -> [actual position].
% During this window, we predict the ball as stationary (vel = 0).
% At 200 Hz with N_hist=100, the guard lasts ~0.55s. The ball hasn't
% traveled far in that time, so Collision Assessment won't miss a threat.
%
% If ball flights are very short and 0.55s is too long, reduce N_hist
% to 20-30 for a faster (but noisier) velocity estimate.

min_samples = int32(opts.N_hist + 10);  % need N_hist clean samples + margin

% ============================================================
% ALWAYS call the velocity estimator so its internal persistent
% history buffer accumulates position samples from the start.
% During the guard window, we just don't trust its output.
% This way, when the guard lifts, the buffer already has
% N_hist clean samples and the first velocity estimate is good.
% ============================================================
vel_opts = struct();
vel_opts.N_hist     = opts.N_hist;
vel_opts.speed_clip = opts.speed_clip;
vel_opts.use_polyfit = true;
vel_est = estimateBallVelocityFromHistory(pos_now, time_now, vel_opts);

if sample_count < min_samples
    vel_est = zeros(3, 1);   % override output, but buffer was populated
end

%% =================== Forward Prediction with Drag ======================
% Integrate the ball trajectory forward using Euler integration with
% quadratic aerodynamic drag.
%
% Physics model:
%   a = g_vec + a_drag
%   a_drag = -drag_coeff * |v| * v     (opposes velocity, quadratic in speed)
%
% This replaces the original closed-form parabolic prediction:
%   x(t) = x0 + vx*t                   (no drag — straight line)
%   z(t) = z0 + vz*t - 0.5*g*t^2       (no drag — parabola)
%
% The Euler integration is necessary because drag makes the ODE
% nonlinear and there is no closed-form solution. At dt = 1/200,
% Euler is stable and accurate enough for prediction purposes.
%
% What we do NOT model:
%   - Magnus force (spin-induced lateral curvature). Would require
%     estimating the spin axis from trajectory curvature, which is
%     not tractable with noisy position-only measurements. Magnus is
%     smaller in magnitude than drag for typical baseball parameters.
%   - Variable gravity (Dynamics.slx uses 0.6g-1.0g). We use standard
%     9.81 m/s^2. The EKF absorbs this mismatch over time.

pos = pos_now;       % initialize integration state: position
vel = vel_est;       % initialize integration state: velocity
dt  = opts.dt;

for k = 1:N_horizon
    tau(k) = (k-1) * dt;

    % Euler step to next timestep (skip on last iteration)
    if k < N_horizon
        speed = norm(vel);

        % Only apply drag if ball is moving (avoid divide-by-zero
        % and spurious drag forces on a near-stationary ball)
        if speed > 0.01
            drag_accel = -drag_coeff * speed * vel;  % opposes velocity
        else
            drag_accel = [0; 0; 0];
        end

        % Total acceleration: gravity + drag (no Magnus)
        accel = g_vec + drag_accel;

        % Forward Euler update
        vel = vel + accel * dt;
        pos = pos + vel * dt;
    end

    % Store current state in output trajectory
    bb_traj(1:3, k) = pos;
    bb_traj(4:6, k) = vel;
end

%% =================== Debug / Diagnostic Outputs ========================
% These scalar outputs are wired to scopes or To Workspace blocks in
% Simulink for quick visual verification.
%   xhat{x,y,z} : the position buildTraj is actually using (should match
%                  the green "actual" line once EKF converges)
%   bb{x,y,z}   : predicted position 1 second ahead (index 200 at 200 Hz)
%   bbv{x,y,z}  : predicted velocity 1 second ahead

xhatx = pos_now(1);
xhaty = pos_now(2);
xhatz = pos_now(3);

bbx  = bb_traj(1, 200);
bby  = bb_traj(2, 200);
bbz  = bb_traj(3, 200);   % check 1s ahead
bbvx = bb_traj(4, 200);
bbvy = bb_traj(5, 200);
bbvz = bb_traj(6, 200);

%% =================== Verbose Debug Output ==============================
if opts.verbose
    fprintf('buildTraj position used: [%g %g %g]\n', ...
        pos_now(1), pos_now(2), pos_now(3));
    fprintf('buildTraj velocity estimated from history: [%g %g %g]\n', ...
        vel_est(1), vel_est(2), vel_est(3));
    fprintf('buildTraj drag_coeff: %g, sample_count: %d\n', ...
        drag_coeff, sample_count);
    % fprintf('velocity estimator method: %s, samples: %d\n', ...
    %     vel_debug.method, vel_debug.numSamples);
end

end
